simulink model "id_manifold_2"  (R2017b)
settings: Solver=VariableStepAuto  StartTime=0.0  StopTime=10.0  RelTol=1e-3
undefined symbols (not defined in the file): pars
settings Model: Creator=emiel  LastModifiedBy=emiel

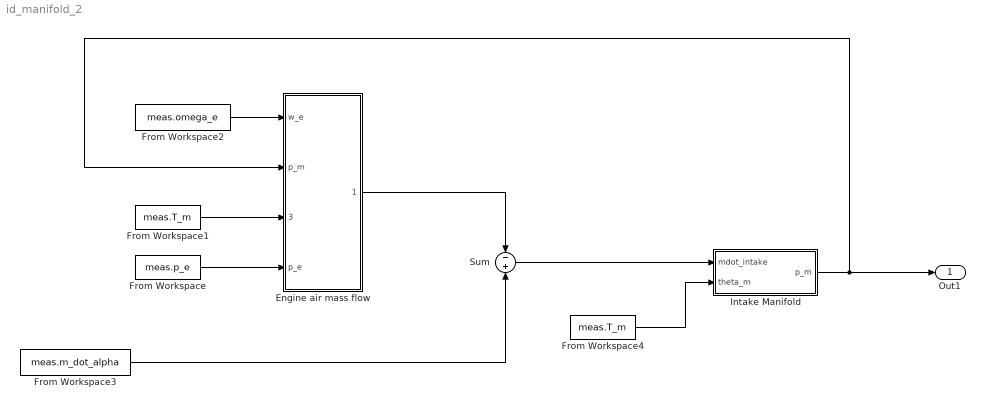
== system id_manifold_2 ==
  Engine air mass flow : Subsystem
  From Workspace : FromWorkspace  VariableName=meas.p_e  SampleTime=0
  From Workspace1 : FromWorkspace  VariableName=meas.T_m  SampleTime=0
  From Workspace2 : FromWorkspace  VariableName=meas.omega_e  SampleTime=0
  From Workspace3 : FromWorkspace  VariableName=meas.m_dot_alpha  SampleTime=0
  From Workspace4 : FromWorkspace  VariableName=meas.T_m  SampleTime=0
  Intake Manifold : Subsystem
  Sum : Sum  Inputs=-|+
  Out1 : Outport
  wires:
  From Workspace/1 -> Engine air mass flow/4(p_e)
  From Workspace1/1 -> Engine air mass flow/3(theta_m)
  Sum/1 -> Intake Manifold/1(mdot_intake)
  Engine air mass flow/1(mdot_beta) -> Sum/1
  From Workspace3/1 -> Sum/2
  From Workspace2/1 -> Engine air mass flow/1(w_e)
  Intake Manifold/1(p_m) -> Engine air mass flow/2(p_m), Out1/1
  From Workspace4/1 -> Intake Manifold/2(theta_m)

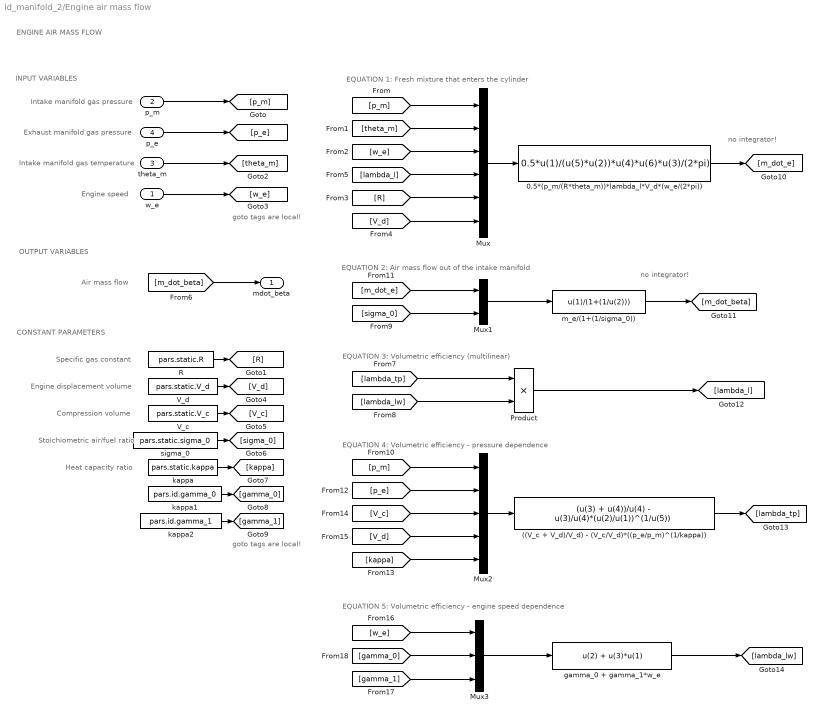
== system id_manifold_2/Engine air mass flow ==
  note: Specific gas constant
  note: Air mass flow
  note: no integrator!
  note: goto tags are local!
  note: CONSTANT PARAMETERS
  note: Stoichiometric air/fuel ratio
  note: INPUT VARIABLES
  note: EQUATION 4: Volumetric efficiency - pressure dependence
  note: Heat capacity ratio
  note: EQUATION 1: Fresh mixture that enters the cylinder
  note: EQUATION 2: Air mass flow out of the intake manifold
  note: goto tags are local!
  note: ENGINE AIR MASS FLOW
  note: no integrator!
  note: EQUATION 5: Volumetric efficiency - engine speed dependence
  note: Intake manifold gas pressure
  note: Exhaust manifold gas pressure
  note: EQUATION 3: Volumetric efficiency (multilinear)
  note: Intake manifold gas temperature
  note: Compression volume
  note: Engine speed
  note: OUTPUT VARIABLES
  note: Engine displacement volume
  w_e : Inport
  p_m : Inport  Port=2
  theta_m : Inport  Port=3
  p_e : Inport  Port=4
  ((V_c + V_d)/V_d) - (V_c/V_d)*((p_e/p_m)^(1/kappa)) : Fcn  Expr=(u(3) + u(4))/u(4) - u(3)/u(4)*(u(2)/u(1))^(1/u(5))
  0.5*(p_m/(R*theta_m))*lambda_l*V_d*(w_e/(2*pi)) : Fcn  Expr=0.5*u(1)/(u(5)*u(2))*u(4)*u(6)*u(3)/(2*pi)
  Mux : Mux  Inputs=6
  Mux1 : Mux  Inputs=2
  Mux2 : Mux  Inputs=5
  Mux3 : Mux  Inputs=3
  Product : Product
  R : Constant  Value=pars.static.R
  V_c : Constant  Value=pars.static.V_c
  V_d : Constant  Value=pars.static.V_d
  gamma_0 + gamma_1*w_e : Fcn  Expr=u(2) + u(3)*u(1)
  kappa : Constant  Value=pars.static.kappa
  kappa1 : Constant  Value=pars.id.gamma_0
  kappa2 : Constant  Value=pars.id.gamma_1
  m_e/(1+(1/sigma_0)) : Fcn  Expr=u(1)/(1+(1/u(2)))
  sigma_0 : Constant  Value=pars.static.sigma_0
  mdot_beta : Outport
  wires:
  kappa/1 -> [kappa]
  [m_dot_beta] -> mdot_beta/1
  [V_d] -> Mux2/4
  [gamma_0] -> Mux3/2
  [w_e] -> Mux3/1
  [p_m] -> Mux2/1
  Mux2/1 -> ((V_c + V_d)/V_d) - (V_c/V_d)*((p_e/p_m)^(1/kappa))/1
  kappa1/1 -> [gamma_0]
  ((V_c + V_d)/V_d) - (V_c/V_d)*((p_e/p_m)^(1/kappa))/1 -> [lambda_tp]
  m_e/(1+(1/sigma_0))/1 -> [m_dot_beta]
  [gamma_1] -> Mux3/3
  w_e/1 -> [w_e]
  Mux3/1 -> gamma_0 + gamma_1*w_e/1
  Mux/1 -> 0.5*(p_m/(R*theta_m))*lambda_l*V_d*(w_e/(2*pi))/1
  [p_m] -> Mux/1
  [m_dot_e] -> Mux1/1
  [V_c] -> Mux2/3
  Product/1 -> [lambda_l]
  p_m/1 -> [p_m]
  [lambda_tp] -> Product/1
  [lambda_l] -> Mux/4
  [R] -> Mux/5
  [lambda_lw] -> Product/2
  [w_e] -> Mux/3
  [V_d] -> Mux/6
  sigma_0/1 -> [sigma_0]
  [theta_m] -> Mux/2
  [sigma_0] -> Mux1/2
  kappa2/1 -> [gamma_1]
  Mux1/1 -> m_e/(1+(1/sigma_0))/1
  p_e/1 -> [p_e]
  V_d/1 -> [V_d]
  [p_e] -> Mux2/2
  gamma_0 + gamma_1*w_e/1 -> [lambda_lw]
  [kappa] -> Mux2/5
  R/1 -> [R]
  V_c/1 -> [V_c]
  0.5*(p_m/(R*theta_m))*lambda_l*V_d*(w_e/(2*pi))/1 -> [m_dot_e]
  theta_m/1 -> [theta_m]

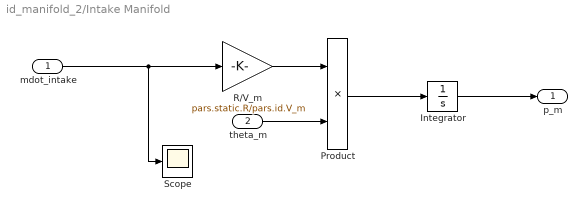
== system id_manifold_2/Intake Manifold ==
  mdot_intake : Inport
  theta_m : Inport  Port=2
  Integrator : Integrator  InitialCondition=pars.init.p_m
  Product : Product
  R/V_m : Gain  Gain=pars.static.R/pars.id.V_m
  Scope : Scope
  p_m : Outport
  wires:
  R/V_m/1 -> Product/1
  theta_m/1 -> Product/2
  Product/1 -> Integrator/1
  Integrator/1 -> p_m/1
  mdot_intake/1 -> R/V_m/1, Scope/1
